simulink model "Tarea5MarioRedondo"  (R2025b)
settings: Solver=VariableStepAuto  StartTime=0.0  StopTime=50  RelTol=1e-3
settings Model: Creator=mredo  LastModifiedBy=mredo

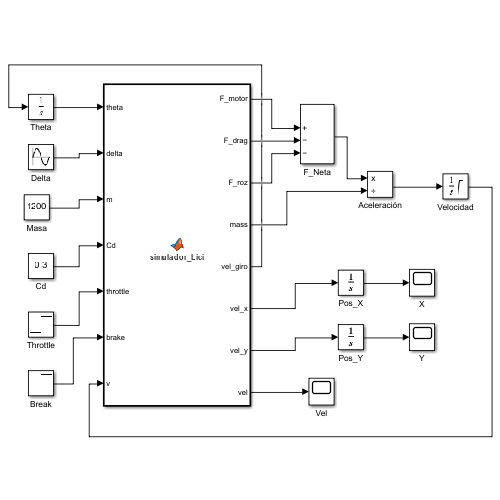
[thumbnail: Simulink's stored preview of the top-level diagram]
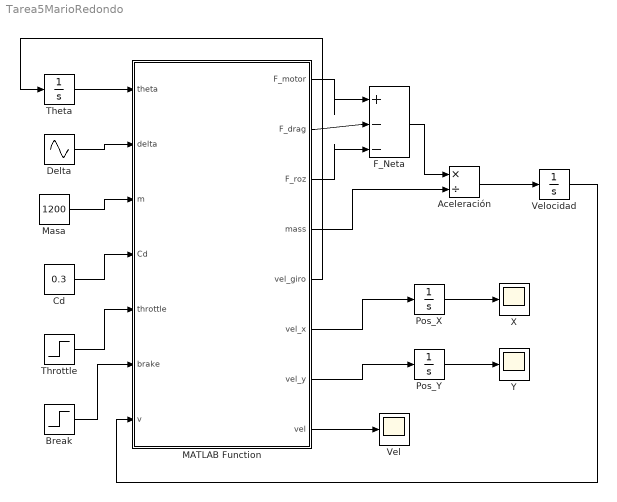
== system Tarea5MarioRedondo ==
  Aceleración : Product  Inputs=*/
  Break : Step  After=0.8  SampleTime=0
  Cd : Constant  Value=0.3
  Delta : Sin  Amplitude=0.2  Frequency=0.5  SampleTime=0
  F_Neta : Sum  Inputs=|+--
  MATLAB Function : MATLAB Function  TreatAsAtomicUnit=on
  Masa : Constant  Value=1200
  Pos_X : Integrator
  Pos_Y : Integrator
  Theta : Integrator
  Throttle : Step  Before=1  After=1.5  SampleTime=0
  Vel : Scope
      settings: ActiveDisplayYMinimum=-1  ActiveDisplayYMaximum=1
  Velocidad : Integrator  LimitOutput=on  LowerSaturationLimit=0
  X : Scope
      settings: ActiveDisplayYMinimum=-37.672083679437613  ActiveDisplayYMaximum=46.150420224127352
  Y : Scope
      settings: ActiveDisplayYMinimum=-53.90694495862234  ActiveDisplayYMaximum=46.212283491304369  DataLoggingVariableName=ScopeData2
  wires:
  Theta/1 -> MATLAB Function/1(theta)
  Throttle/1 -> MATLAB Function/5(throttle)
  Break/1 -> MATLAB Function/6(brake)
  MATLAB Function/1(F_motor) -> F_Neta/1
  MATLAB Function/2(F_drag) -> F_Neta/2
  MATLAB Function/3(F_roz) -> F_Neta/3
  F_Neta/1 -> Aceleración/1
  MATLAB Function/4(mass) -> Aceleración/2
  Aceleración/1 -> Velocidad/1
  Velocidad/1 -> MATLAB Function/7(v)
  MATLAB Function/5(vel_giro) -> Theta/1
  Delta/1 -> MATLAB Function/2(delta)
  Masa/1 -> MATLAB Function/3(m)
  Cd/1 -> MATLAB Function/4(Cd)
  MATLAB Function/8(vel) -> Vel/1
  MATLAB Function/6(vel_x) -> Pos_X/1
  MATLAB Function/7(vel_y) -> Pos_Y/1
  Pos_Y/1 -> Y/1
  Pos_X/1 -> X/1

== matlab function Tarea5MarioRedondo/MATLAB Function ==
  data: F_motor output; F_drag output; F_roz output; mass output; vel_giro output; vel_x output; vel_y output; theta input; delta input; m input; Cd input; throttle input; brake input; v input; vel output
function [F_motor, F_drag, F_roz, mass, vel_giro, vel_x, vel_y, vel] =  simulador_bici(theta, delta, m, Cd, throttle, brake, v)
    %%Parametros constantes
    A=2.2; %Area frontal (m^2)
    p = 1.225; %Densidad del aire
    L = 2.5; %Longitud entre los ejes (m)
    g = 9.8; %Gravedad (N * kg^-1)
    mu = 0.02; %Coeficiente de rozamiento
    
    %%Fuerzas
    %Fuerza del motor y freno
    %Ponemos (800*brake) para que al frenar si se pueda frenar el coche y no
    %sea un sinsentido ya que si no lo ponemos le costará un mundo frenar
    F_motor = (m*throttle) - (800*brake);
    
    %Fuerza aerodinámica
    F_drag = 0.5 * p * Cd * A * v^2;
    
    %Fuerza rozamiento
    F_roz = mu * m * g;

    %%Masa
    mass = m;
    
    %%Velocidades
    vel_giro = (v / L) * tan(delta);
    vel_x = v * cos(theta);
    vel_y = v * sin(theta);
    vel = v;
end
